simulink model "LeadController"  (R2021b)
settings: Solver=VariableStepAuto  StartTime=0.0  StopTime=20  RelTol=1e-3
model workspace (MAT data in the model file):
  L = 0.2
values from neighbouring files (symbols this model uses):
  Td = 100e-6    (= 0.0001)    [simConstants.m]
libraries: simulink_extras x1
settings Model: Creator=logan  LastModifiedBy=logan

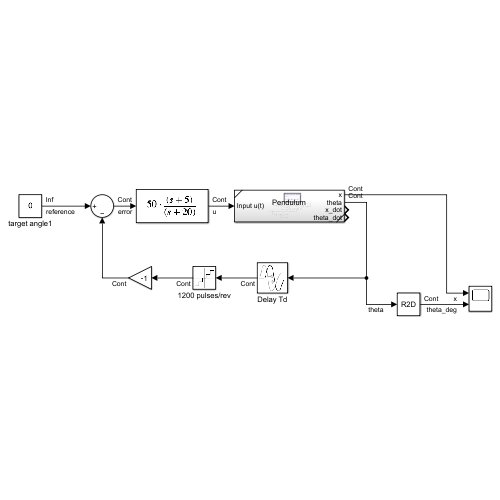
[thumbnail: Simulink's stored preview of the top-level diagram]
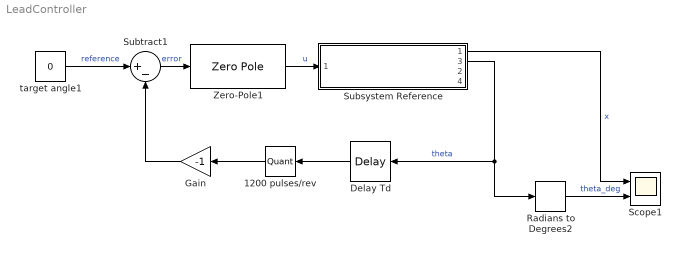
== system LeadController ==
  1200 pulses/rev : Quantizer  QuantizationInterval=(2*pi)/1200
  Delay Td : TransportDelay  DelayTime=Td*10
  Gain : Gain  Gain=-1
  Radians to Degrees2 : simulink_extras/Transformations/Radians to Degrees
  Scope1 : Scope  NumInputPorts=2
  Subsystem Reference : Subsystem  ReferencedSubsystem=Pendulum
      settings: PortSchema="{\"entries\":[{\"content\":{\"sides\":[{\"content\":{\"connectorIds\":[\"In1\"]},\"type\":\"ConnectorPlacement.EquallySpacedRectSide\",\"uuid\":\"caec1104-e2e6-4c31-8105-8fc922dae5e8\"},{\"content\":{\"connectorIds\":[\"Out1\",\"Out3\",\"Out2\",\"Out4\"],\"side\":\"RIGHT\"},\"type\":\"ConnectorPlacement.EquallySpacedRectSide\",\"uuid\":\"5fd37d83-c645-402c-ac25-1888ccf1b1a6\"},{\"content\":{\"connectorIds\":[],\"side\":\"TOP\"},\"type\":\"ConnectorPlacement.EquallySpacedRectSide\",\"uuid\":\"2e43f1c0-40e6-4dcf-a44e-f71c6f7202b4\"}]},\"type\":\"ConnectorPlacement.EquallySpacedConnector\",\"uuid\":\"6200bc17-7860-41df-9508-8c7d9814e84e\"}],\"packageUris\":[\"http://schema.mathworks.com/mf0/Connector/R2020b\"],\"version\":\"1.0\"}"
  Subtract1 : Sum  Inputs=|+-
  Zero-Pole1 : ZeroPole  Zeros=-5  Poles=-20  Gain=50
  target angle1 : Constant  Value=0  OutDataTypeStr=Inherit: Inherit via back propagation
  wires:
  Radians to Degrees2/1 -> Scope1/2  "theta_deg"
  Gain/1 -> Subtract1/2
  Subsystem Reference/1 -> Scope1/1  "x"
  Zero-Pole1/1 -> Subsystem Reference/1  "u"
  Subsystem Reference/3 -> Delay Td/1, Radians to Degrees2/1  "theta"
  target angle1/1 -> Subtract1/1  "reference"
  Subtract1/1 -> Zero-Pole1/1  "error"
  Delay Td/1 -> 1200 pulses/rev/1
  1200 pulses/rev/1 -> Gain/1
